simulink subsystem "LinerizePi18"  (R2023a)
settings: Solver=VariableStepAuto  StartTime=0.0  StopTime=10.0  RelTol=1e-3
settings Model: Creator=ycheb  LastModifiedBy=ycheb

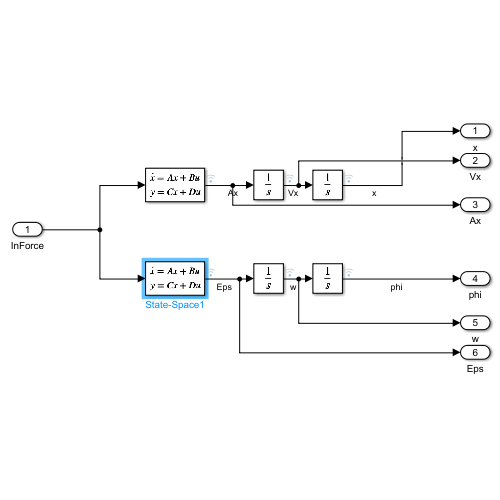
[thumbnail: Simulink's stored preview of the top-level diagram]
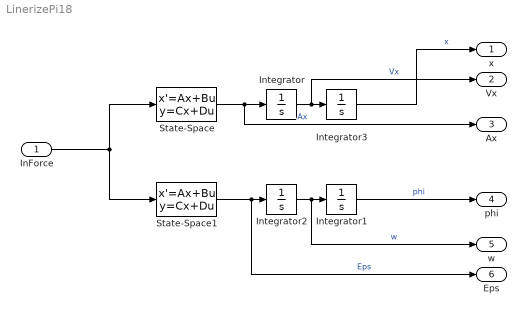
== system LinerizePi18 ==
  InForce : Inport
  Integrator : Integrator
  Integrator1 : Integrator  InitialCondition=-5*pi/180
  Integrator2 : Integrator
  Integrator3 : Integrator
  State-Space : StateSpace  A="[1\t0\t0\t-0.00326633498892640;0.00100000000000000\t1\t0\t-1.63316749446320e-06;0\t0\t1.00000367486232\t0.00979939010085565;0\t0\t0.00100000122495381\t1.00000489969205]"  B=[0.004444331628905;2.222165814452640e-06;-0.003333125884701;-1.666561921620334e-06]  C=[0,0,0,-3.266334988926396]  D=4.444331628905281  InitialCondition=0
  State-Space1 : StateSpace  A="[1\t0\t0\t-0.00326633498892640;0.00100000000000000\t1\t0\t-1.63316749446320e-06;0\t0\t1.00000367486232\t0.00979939010085565;0\t0\t0.00100000122495381\t1.00000489969205]"  B=[0.004444331628905;2.222165814452640e-06;-0.003333125884701;-1.666561921620334e-06]  C=[0,0,0,9.799378097070152]  D=-3.333121801780800  InitialCondition=0
  x : Outport
  Vx : Outport  Port=2
  Ax : Outport  Port=3
  phi : Outport  Port=4
  w : Outport  Port=5
  Eps : Outport  Port=6
  wires:
  Integrator/1 -> Vx/1, Integrator3/1  "Vx"
  Integrator3/1 -> x/1  "x"
  Integrator2/1 -> w/1, Integrator1/1  "w"
  Integrator1/1 -> phi/1  "phi"
  State-Space1/1 -> Eps/1, Integrator2/1  "Eps"
  State-Space/1 -> Ax/1, Integrator/1  "Ax"
  InForce/1 -> State-Space1/1, State-Space/1
